simulink model "Simulation_Model_Env"  (R2024a)
settings: Solver=ode45  StartTime=0  StopTime=inf  FixedStep=0.001  MaxStep=0.1  RelTol=1e-6  AbsTol=1e-6  EnableMultiTasking=on
values from neighbouring files (symbols this model uses):
  batteryCap = 1000    [trainingData.mat]
  IrrData10pcLow = [1233 1234 1569 1570 1688 1689 4307 3623 1156 1118 1161 3247 ... (547 elements, 1x547)]    [trainingData.mat]
  pvCap = 1300    [trainingData.mat]
undefined symbols (not defined in the file or in its folder): seedDay, timeEpisode
libraries: simulink x8, rllib x1
settings Model: Creator=feliz  LastModifiedBy=bretz68
settings SolverCC: AutoScaleAbsTol=off  ZeroCrossControl=DisableAll
settings DataIOCC: LimitDataPoints=on  SaveFormat=Array
settings OptimizationCC: ExpressionDepthLimit=2147483647  LifeSpan=inf
settings DebuggingCC: UnderspecifiedInitializationDetection=Classic  MergeDetectMultiDrivingBlocksExec=none  SolverPrmCheckMsg=warning  UnconnectedInputMsg=warning  UnconnectedOutputMsg=warning  UnconnectedLineMsg=warning  AllowSymbolicDim=off  StateNameClashWarn=warning  SFUnexpectedBacktrackingDiag=warning  SFNoUnconditionalDefaultTransitionDiag=warning  SFExecutionAtInitializationDiag=none  ArithmeticOperatorsInVariantConditions=warning
settings HardwareCC: ProdBitPerPointer=32  ProdBitPerSizeT=32  ProdBitPerPtrDiffT=32  ProdLargestAtomicFloat=None  ProdIntDivRoundTo=Undefined  ProdEndianess=Unspecified  ProdWordSize=32  ProdHWDeviceType=32-bit Generic
settings ModelReferenceCC: EnableRefExpFcnMdlSchedulingChecks=on  PropagateSignalLabelsOutOfModel=off
settings SFSimCC: SimUseLocalCustomCode=off  CustomCodeUndefinedFunction=UseInterfaceOnly
settings RTWCC: RTWUseLocalCustomCode=off  GPUComputeCapability=3.5
settings CodeAppCC: StateflowObjectComments=on
settings GRTTargetCC: TargetLangStandard=C89/C90 (ANSI)
settings ConfigComp: CovMetricSettings=dw  CovSaveCumulativeToWorkspaceVar=on  CovSaveSingleToWorkspaceVar=on  CovExternalEMLEnable=off

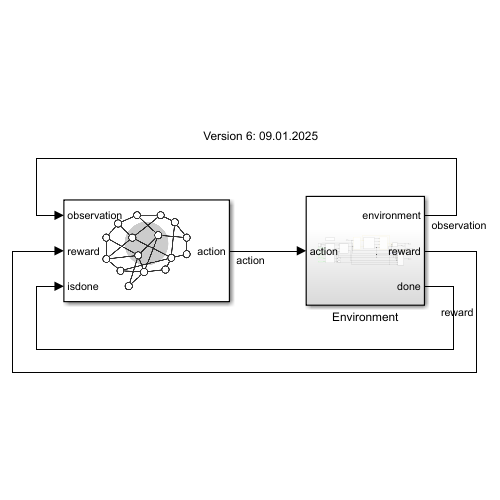
[thumbnail: Simulink's stored preview of the top-level diagram]
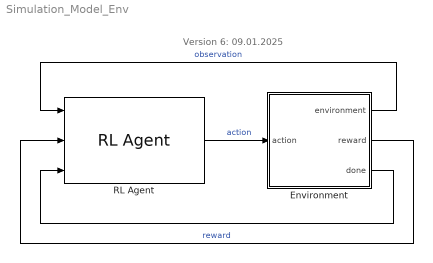
== system Simulation_Model_Env ==
  note: Version 6: 09.01.2025
  Environment : Subsystem
  RL Agent : rllib/RL Agent  Agent=ppoRealAgentv10  ExternalActionAsInput=off  ProvideLastAction=off  ProvideCumRwd=off  TreatAsDirectFeedthrough=on  UseStrictObservationDataTypes=off
  wires:
  Environment/1(environment) -> RL Agent/1  "observation"
  RL Agent/1 -> Environment/1(action)  "action"
  Environment/2(reward) -> RL Agent/2  "reward"
  Environment/3(done) -> RL Agent/3

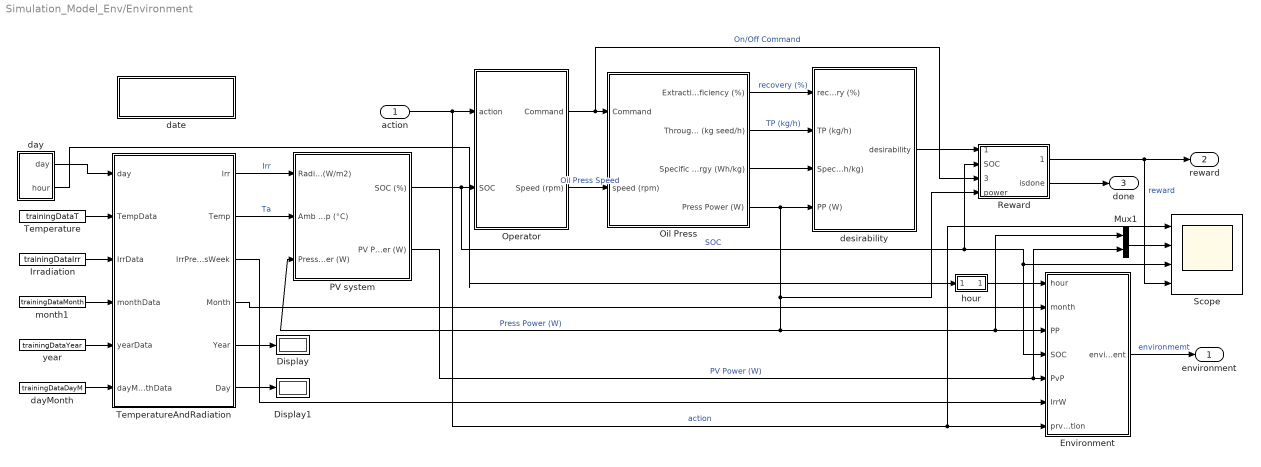
== system Simulation_Model_Env/Environment ==
  action : Inport
  Display : Display
  Display1 : Display
  Environment : Subsystem
  Irradiation : FromWorkspace  VariableName=trainingDataIrr  OutDataTypeStr=double  SampleTime=timeEpisode+1
  Mux1 : Mux  Inputs=2
  Oil Press : Subsystem
  Operator : Subsystem
  PV system : Subsystem
  Reward : Subsystem
  Scope : Scope  NumInputPorts=4
  Temperature : FromWorkspace  VariableName=trainingDataT  OutDataTypeStr=double  SampleTime=timeEpisode+1
  TemperatureAndRadiation : MATLAB Function  TreatAsAtomicUnit=on
  date : Subsystem
  day : Subsystem
  dayMonth : FromWorkspace  VariableName=trainingDataDayM  OutDataTypeStr=double  SampleTime=timeEpisode+1
  desirability : Subsystem
  hour : Subsystem
  month1 : FromWorkspace  VariableName=trainingDataMonth  OutDataTypeStr=double  SampleTime=timeEpisode+1
  year : FromWorkspace  VariableName=trainingDataYear  OutDataTypeStr=double  SampleTime=timeEpisode+1
  environment : Outport
  reward : Outport  Port=2
  done : Outport  Port=3
  wires:
  TemperatureAndRadiation/2(Temp) -> PV system/2(Amb Temp (°C))  "Ta"
  Operator/1("Command ") -> Reward/3(command), Oil Press/1(Command)  "On/Off Command"
  Irradiation/1 -> TemperatureAndRadiation/3(IrrData)
  TemperatureAndRadiation/1(Irr) -> PV system/1(Radiation on Surf (W/m2))  "Irr"
  Temperature/1 -> TemperatureAndRadiation/2(TempData)
  Oil Press/2(Throughput (kg seed/h)) -> desirability/2(TP (kg/h))  "TP (kg/h)"
  Operator/2(Speed (rpm)) -> Oil Press/2(speed (rpm))  "Oil Press Speed"
  Oil Press/1(Extraction Efficiency (%)) -> desirability/1(recovery (%))  "recovery (%)"
  desirability/1(desirability) -> Reward/1(desirability)
  Oil Press/3(Specific energy (Wh/kg)) -> desirability/3(Spec Enr (Wh/kg))
  TemperatureAndRadiation/3(IrrPreviousWeek) -> Environment/6(IrrW)
  hour/1(hour) -> Environment/1(hour)
  day/1(day) -> TemperatureAndRadiation/1(day)
  Reward/2(isdone) -> done/1
  Environment/1(environment) -> environment/1  "environmemt"
  month1/1 -> TemperatureAndRadiation/4(monthData)
  TemperatureAndRadiation/4(Month) -> Environment/2(month)
  PV system/1(SOC (%)) -> Environment/4(SOC), Scope/3, Reward/2(SOC), Operator/2(SOC)  "SOC"
  Mux1/1 -> Scope/2
  action/1 -> Operator/1(action), Environment/7(prvAction), Scope/1  "action"
  Reward/1(reward) -> Scope/4, reward/1  "reward"
  Oil Press/4("Press Power (W) ") -> desirability/4(PP (W)), Reward/4(power), Environment/3(PP), Mux1/1, PV system/3(Press Power (W))  "Press Power (W)"
  PV system/2(PV Power (W)) -> Mux1/2, Environment/5(PvP)  "PV Power (W)"
  year/1 -> TemperatureAndRadiation/5(yearData)
  TemperatureAndRadiation/5(Year) -> Display/1
  TemperatureAndRadiation/6(Day) -> Display1/1
  dayMonth/1 -> TemperatureAndRadiation/6(dayMonthData)
  day/2(hour) -> hour/1(simhour)

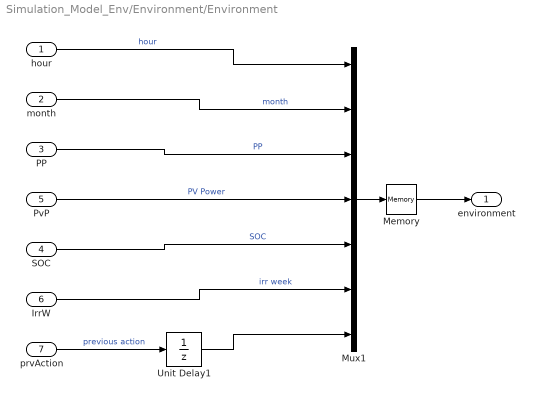
== system Simulation_Model_Env/Environment/Environment ==
  hour : Inport
  month : Inport  Port=2
  PP : Inport  Port=3
  SOC : Inport  Port=4
  PvP : Inport  Port=5
  IrrW : Inport  Port=6
  prvAction : Inport  Port=7
  Memory : Memory
  Mux1 : Mux  Inputs=7
  Unit Delay1 : UnitDelay  SampleTime=-1  HasFrameUpgradeWarning=on
  environment : Outport
  wires:
  SOC/1 -> Mux1/5  "SOC"
  PvP/1 -> Mux1/4  "PV Power"
  IrrW/1 -> Mux1/6  "irr week"
  hour/1 -> Mux1/1  "hour"
  PP/1 -> Mux1/3  "PP"
  month/1 -> Mux1/2  "month"
  Mux1/1 -> Memory/1
  prvAction/1 -> Unit Delay1/1  "previous action"
  Unit Delay1/1 -> Mux1/7
  Memory/1 -> environment/1

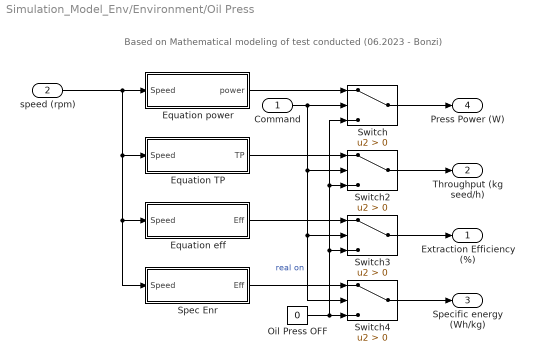
== system Simulation_Model_Env/Environment/Oil Press ==
  note: Based on Mathematical modeling of test conducted (06.2023 - Bonzi)
  Command : Inport
  speed (rpm) : Inport  Port=2
  Equation TP : Subsystem
  Equation eff : Subsystem
  Equation power : Subsystem
  Oil Press OFF : Constant  Value=0
  Spec Enr : Subsystem
  Switch{,2..4} (4 alike) : Switch  Criteria=u2 > Threshold  SaturateOnIntegerOverflow=off  InputSameDT=off
  Extraction Efficiency (%) : Outport
  Throughput (kg seed/h) : Outport  Port=2
  Specific energy (Wh/kg) : Outport  Port=3
  "Press Power (W) " : Outport  Port=4
  wires:
  Switch3/1 -> Extraction Efficiency (%)/1
  Switch/1 -> "Press Power (W) "/1
  Equation power/1(power) -> Switch/1
  Equation TP/1(TP) -> Switch2/1
  Switch2/1 -> Throughput (kg seed/h)/1
  Equation eff/1(Eff) -> Switch3/1
  Oil Press OFF/1 -> Switch3/3, Switch2/3, Switch/3, Switch4/3
  speed (rpm)/1 -> Spec Enr/1(Speed), Equation eff/1(Speed), Equation TP/1(Speed), Equation power/1(Speed)
  Command/1 -> Switch4/2, Switch3/2, Switch2/2, Switch/2  "real on"
  Switch4/1 -> Specific energy (Wh/kg)/1
  Spec Enr/1(Eff) -> Switch4/1

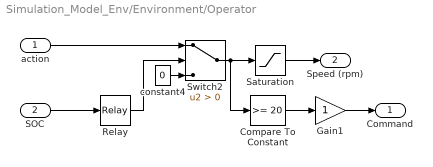
== system Simulation_Model_Env/Environment/Operator ==
  action : Inport
  SOC : Inport  Port=2
  Compare To Constant : simulink/Logic and Bit Operations/Compare To Constant  relop=>=  const=20  OutDataTypeStr=boolean
  Gain1 : Gain  OutDataTypeStr=double
  Relay : Relay  OnSwitchValue=25  OffSwitchValue=20
  Saturation : Saturate  UpperLimit=70  LowerLimit=0
  Switch2 : Switch  Criteria=u2 > Threshold  SaturateOnIntegerOverflow=off  InputSameDT=off
  constant4 : Constant  Value=0
  "Command " : Outport
  Speed (rpm) : Outport  Port=2
  wires:
  SOC/1 -> Relay/1
  Switch2/1 -> Compare To Constant/1, Saturation/1
  Relay/1 -> Switch2/2
  action/1 -> Switch2/1
  constant4/1 -> Switch2/3
  Compare To Constant/1 -> Gain1/1
  Saturation/1 -> Speed (rpm)/1
  Gain1/1 -> "Command "/1

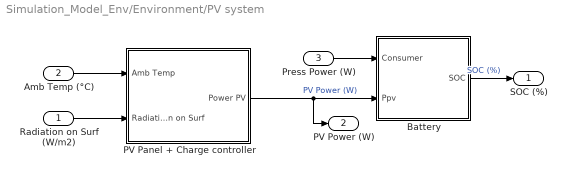
== system Simulation_Model_Env/Environment/PV system ==
  Radiation on Surf (W/m2) : Inport
  Amb Temp (°C) : Inport  Port=2
  Press Power (W) : Inport  Port=3
  Battery : Subsystem
      mask Display: image('bat.PNG'); % Use "Edit Image" on toolstrip to change.
  PV Panel + Charge controller : Subsystem
      mask Display: image('pvmppt.PNG'); % Use "Edit Image" on toolstrip to change.
  SOC (%) : Outport
  PV Power (W) : Outport  Port=2
  wires:
  Amb Temp (°C)/1 -> PV Panel + Charge controller/1(Amb Temp)
  PV Panel + Charge controller/1(Power PV) -> PV Power (W)/1, Battery/2(Ppv)  "PV Power (W)"
  Press Power (W)/1 -> Battery/1(Consumer)
  Battery/1(SOC) -> SOC (%)/1  "SOC (%)"
  Radiation on Surf (W/m2)/1 -> PV Panel + Charge controller/2(Radiation on Surf)

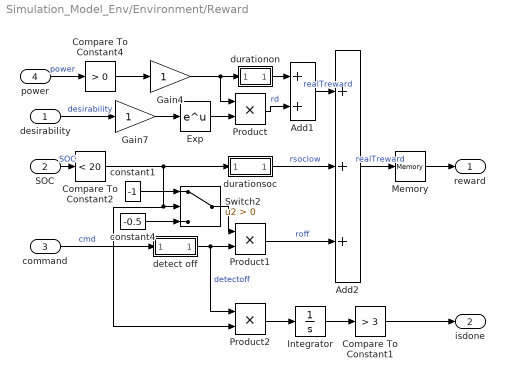
== system Simulation_Model_Env/Environment/Reward ==
  desirability : Inport
  SOC : Inport  Port=2
  command : Inport  Port=3
  power : Inport  Port=4
  Add1 : Sum
  Add2 : Sum  Inputs=+++
  Compare To Constant1 : simulink/Logic and Bit Operations/Compare To Constant  relop=>  const=3  OutDataTypeStr=boolean
  Compare To Constant2 : simulink/Logic and Bit Operations/Compare To Constant  relop=<  const=20  OutDataTypeStr=boolean
  Compare To Constant4 : simulink/Logic and Bit Operations/Compare To Constant  relop=>  const=0  OutDataTypeStr=boolean
  Exp : Math
  Gain4 : Gain  OutDataTypeStr=double
  Gain7 : Gain  OutDataTypeStr=double
  Integrator : Integrator
  Memory : Memory
  Product : Product
  Product1 : Product
  Product2 : Product  OutDataTypeStr=double
  Switch2 : Switch  Criteria=u2 > Threshold  SaturateOnIntegerOverflow=off  InputSameDT=off
  constant1 : Constant  Value=-1
  constant4 : Constant  Value=-0.5
  detect off : Subsystem
  durationon : Subsystem
  durationsoc : Subsystem
  reward : Outport
  isdone : Outport  Port=2
  wires:
  desirability/1 -> Gain7/1  "desirability"
  Gain7/1 -> Exp/1
  durationsoc/1(Out1) -> Add2/2  "rsoclow"
  Add2/1 -> Memory/1  "realTreward"
  Exp/1 -> Product/2
  Memory/1 -> reward/1
  detect off/1(Out1) -> Product2/1, Product1/2  "detectoff"
  command/1 -> detect off/1(cmd)  "cmd"
  Product1/1 -> Add2/3  "roff"
  SOC/1 -> Compare To Constant2/1  "SOC"
  Compare To Constant4/1 -> Gain4/1
  Gain4/1 -> durationon/1(on), Product/1
  Product/1 -> Add1/2  "rd"
  constant4/1 -> Switch2/3
  constant1/1 -> Switch2/1
  Switch2/1 -> Product1/1
  power/1 -> Compare To Constant4/1  "power"
  Compare To Constant2/1 -> durationsoc/1(isco), Product2/2, Switch2/2
  Add1/1 -> Add2/1  "realTreward"
  durationon/1(Out1) -> Add1/1
  Integrator/1 -> Compare To Constant1/1
  Compare To Constant1/1 -> isdone/1
  Product2/1 -> Integrator/1

== system Simulation_Model_Env/Environment/date ==
  note: /
  note: Date
  note: /
  Display1 : DisplayBlock  LabelPosition=Hide  Transparency=1
  Display2 : DisplayBlock  LabelPosition=Hide  Transparency=1  ShowGrid=off
  Display3 : DisplayBlock  LabelPosition=Hide  Transparency=1  ShowGrid=off

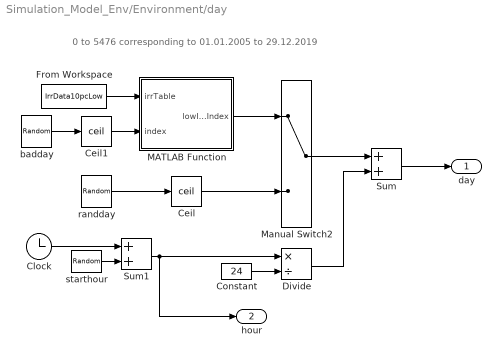
== system Simulation_Model_Env/Environment/day ==
  note: 0 to 5476 corresponding to 01.01.2005 to 29.12.2019
  Ceil : Rounding  Operator=ceil
  Ceil1 : Rounding  Operator=ceil
  Clock : Clock
  Constant : Constant  Value=24
  Divide : Product  Inputs=*/
  From Workspace : FromWorkspace  VariableName=IrrData10pcLow  SampleTime=timeEpisode+1
  MATLAB Function : MATLAB Function  TreatAsAtomicUnit=on
  Manual Switch2 : ManualSwitch
  Sum : Sum
  Sum1 : Sum
  badday : UniformRandomNumber  Minimum=0  Maximum=length(IrrData10pcLow)-1  Seed=seedDay  SampleTime=timeEpisode+1
  randday : UniformRandomNumber  Minimum=0  Maximum=5476  Seed=seedDay  SampleTime=timeEpisode+1
  starthour : UniformRandomNumber  Minimum=0  Maximum=23  Seed=seedDay  SampleTime=timeEpisode+1
  day : Outport
  hour : Outport  Port=2
  wires:
  randday/1 -> Ceil/1
  Ceil/1 -> Manual Switch2/2
  Constant/1 -> Divide/2
  Clock/1 -> Sum1/1
  Divide/1 -> Sum/2
  Sum/1 -> day/1
  From Workspace/1 -> MATLAB Function/1(irrTable)
  MATLAB Function/1(lowIrrDayIndex) -> Manual Switch2/1
  Manual Switch2/1 -> Sum/1
  starthour/1 -> Sum1/2
  Sum1/1 -> hour/1, Divide/1
  badday/1 -> Ceil1/1
  Ceil1/1 -> MATLAB Function/2(index)

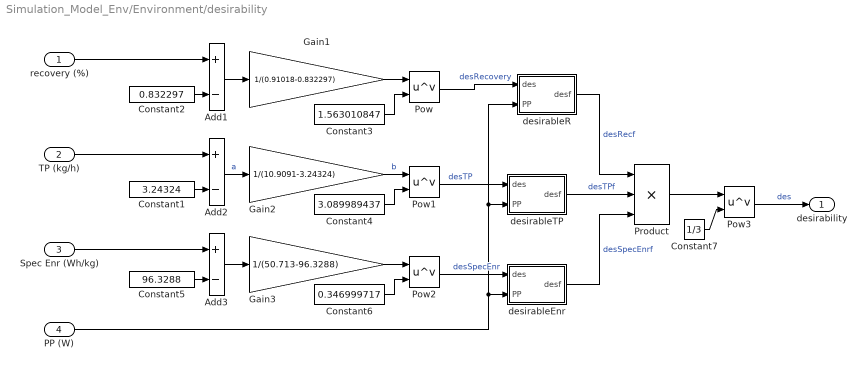
== system Simulation_Model_Env/Environment/desirability ==
  recovery (%) : Inport
  TP (kg/h) : Inport  Port=2
  Spec Enr (Wh/kg) : Inport  Port=3
  PP (W) : Inport  Port=4
  Add1 : Sum  Inputs=+-
  Add2 : Sum  Inputs=+-
  Add3 : Sum  Inputs=+-
  Constant1 : Constant  Value=3.24324
  Constant2 : Constant  Value=0.832297
  Constant3 : Constant  Value=1.563010847
  Constant4 : Constant  Value=3.089989437
  Constant5 : Constant  Value=96.3288
  Constant6 : Constant  Value=0.346999717
  Constant7 : Constant  Value=1/3
  Gain1 : Gain  Gain=1/(0.91018-0.832297)
  Gain2 : Gain  Gain=1/(10.9091-3.24324)
  Gain3 : Gain  Gain=1/(50.713-96.3288)
  Pow{,1..3} (4 alike) : Math  Operator=pow  SignedPower=on  RndMeth=Zero
  Product : Product  Inputs=3
  desirableEnr : Subsystem
  desirableR : Subsystem
  desirableTP : Subsystem
  desirability : Outport
  wires:
  Add1/1 -> Gain1/1
  recovery (%)/1 -> Add1/1
  Constant2/1 -> Add1/2
  Gain1/1 -> Pow/1
  Constant3/1 -> Pow/2
  Constant1/1 -> Add2/2
  Gain2/1 -> Pow1/1  "b"
  Constant4/1 -> Pow1/2
  Add2/1 -> Gain2/1  "a"
  TP (kg/h)/1 -> Add2/1
  Add3/1 -> Gain3/1
  Gain3/1 -> Pow2/1
  Constant5/1 -> Add3/2
  Constant6/1 -> Pow2/2
  Spec Enr (Wh/kg)/1 -> Add3/1
  Product/1 -> Pow3/1
  desirableTP/1(desf) -> Product/2  "desTPf"
  desirableEnr/1(desf) -> Product/3  "desSpecEnrf"
  Pow/1 -> desirableR/1(des)  "desRecovery"
  desirableR/1(desf) -> Product/1  "desRecf"
  Pow1/1 -> desirableTP/1(des)  "desTP"
  Pow2/1 -> desirableEnr/1(des)  "desSpecEnr"
  PP (W)/1 -> desirableR/2(PP), desirableTP/2(PP), desirableEnr/2(PP)
  Constant7/1 -> Pow3/2
  Pow3/1 -> desirability/1  "des"

== system Simulation_Model_Env/Environment/hour ==
  simhour : Inport
  Constant : Constant  Value=24
  Mod : Math  Operator=mod
  hour : Outport
  wires:
  simhour/1 -> Mod/1
  Mod/1 -> hour/1
  Constant/1 -> Mod/2

== system Simulation_Model_Env/Environment/Oil Press/Equation TP ==
  Speed : Inport
  Add : Sum  Inputs=+++
  Gain1 : Gain  Gain=0.217737397
  Product : Product  Inputs=3
  constant : Constant  Value=-0.000675351
  constant4 : Constant  Value=-0.998344774
  TP : Outport
  wires:
  Gain1/1 -> Add/2
  Product/1 -> Add/3
  constant/1 -> Product/3
  constant4/1 -> Add/1
  Speed/1 -> Gain1/1, Product/2, Product/1
  Add/1 -> TP/1

== system Simulation_Model_Env/Environment/Oil Press/Equation eff ==
  Speed : Inport
  Add : Sum  Inputs=+++
  Gain1 : Gain  Gain=-0.003110656
  Product : Product  Inputs=3
  constant : Constant  Value=2.56866E-05
  constant4 : Constant  Value=0.95370599
  Eff : Outport
  wires:
  Gain1/1 -> Add/2
  Product/1 -> Add/3
  constant/1 -> Product/3
  constant4/1 -> Add/1
  Speed/1 -> Product/2, Product/1, Gain1/1
  Add/1 -> Eff/1

== system Simulation_Model_Env/Environment/Oil Press/Equation power ==
  Speed : Inport
  Add : Sum  Inputs=+++
  Gain1 : Gain  Gain=8.7
  Product : Product  Inputs=3
  constant : Constant  Value=-0.05
  constant4 : Constant  Value=57.3
  power : Outport
  wires:
  Gain1/1 -> Add/2
  Product/1 -> Add/3
  constant/1 -> Product/3
  constant4/1 -> Add/1
  Speed/1 -> Gain1/1, Product/2, Product/1
  Add/1 -> power/1

== system Simulation_Model_Env/Environment/Oil Press/Spec Enr ==
  Speed : Inport
  Add : Sum  Inputs=+++
  Gain1 : Gain  Gain=-0.977028804
  Product : Product  Inputs=3
  constant : Constant  Value=0.004169482
  constant4 : Constant  Value=97.14879537
  Eff : Outport
  wires:
  Gain1/1 -> Add/2
  Product/1 -> Add/3
  constant/1 -> Product/3
  constant4/1 -> Add/1
  Speed/1 -> Product/2, Product/1, Gain1/1
  Add/1 -> Eff/1

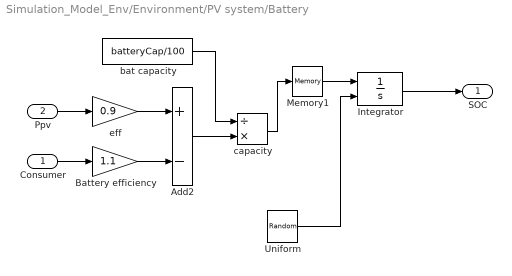
== system Simulation_Model_Env/Environment/PV system/Battery ==
  Consumer : Inport
  Ppv : Inport  Port=2
  Add2 : Sum  Inputs=+-
  Battery efficiency : Gain  Gain=1.1
  Integrator : Integrator  InitialConditionSource=external  InitialCondition=20  LimitOutput=on  UpperSaturationLimit=100  LowerSaturationLimit=0
  Memory1 : Memory
  Uniform : UniformRandomNumber  Minimum=20  Maximum=100  Seed=seedDay  SampleTime=timeEpisode+1
  bat capacity : Constant  Value=batteryCap/100
  capacity : Product  Inputs=/*
  eff : Gain  Gain=0.9
  SOC : Outport
  wires:
  Ppv/1 -> eff/1
  Consumer/1 -> Battery efficiency/1
  capacity/1 -> Memory1/1
  Add2/1 -> capacity/2
  bat capacity/1 -> capacity/1
  eff/1 -> Add2/1
  Battery efficiency/1 -> Add2/2
  Integrator/1 -> SOC/1
  Uniform/1 -> Integrator/2
  Memory1/1 -> Integrator/1

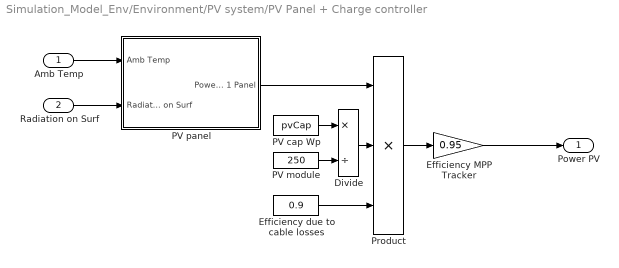
== system Simulation_Model_Env/Environment/PV system/PV Panel + Charge controller ==
  Amb Temp : Inport
  Radiation on Surf : Inport  Port=2
  Divide : Product  Inputs=*/
  Efficiency MPP Tracker : Gain  Gain=0.95
  Efficiency due to cable losses : Constant  Value=0.9
  PV cap Wp : Constant  Value=pvCap
  PV module : Constant  Value=250
  PV panel : Subsystem
  Product : Product  Inputs=3  RndMeth=Zero
  Power PV : Outport
  wires:
  Product/1 -> Efficiency MPP Tracker/1
  Efficiency MPP Tracker/1 -> Power PV/1
  PV panel/1(Power PV 1 Panel) -> Product/1
  PV cap Wp/1 -> Divide/1
  Efficiency due to cable losses/1 -> Product/3
  Amb Temp/1 -> PV panel/1(Amb Temp)
  Radiation on Surf/1 -> PV panel/2(Radiation on Surf)
  Divide/1 -> Product/2
  PV module/1 -> Divide/2

== system Simulation_Model_Env/Environment/Reward/detect off ==
  cmd : Inport
  Add : Sum  Inputs=+-
  Compare To Constant : simulink/Logic and Bit Operations/Compare To Constant  relop=<  const=0  OutDataTypeStr=boolean
  Unit Delay : UnitDelay  SampleTime=-1  HasFrameUpgradeWarning=on
  Out1 : Outport
  wires:
  Add/1 -> Compare To Constant/1
  Unit Delay/1 -> Add/2  "cmdDel"
  cmd/1 -> Unit Delay/1, Add/1  "cmd"
  Compare To Constant/1 -> Out1/1  "intdiff"

== system Simulation_Model_Env/Environment/Reward/durationon ==
  on : Inport
  Add : Sum
  Gain3 : Gain  Gain=0.01  OutDataTypeStr=double
  Memory : Memory
  Product : Product
  Out1 : Outport
  wires:
  Add/1 -> Product/2
  Memory/1 -> Add/2
  Gain3/1 -> Add/1
  on/1 -> Product/1, Gain3/1
  Product/1 -> Memory/1, Out1/1

== system Simulation_Model_Env/Environment/Reward/durationsoc ==
  isco : Inport
  Add : Sum
  Gain1 : Gain  Gain=-1  OutDataTypeStr=double
  Gain3 : Gain  Gain=0.02  OutDataTypeStr=double
  Memory : Memory
  Product : Product
  Out1 : Outport
  wires:
  Add/1 -> Product/2
  Memory/1 -> Add/2
  Gain3/1 -> Add/1
  Product/1 -> Memory/1, Gain1/1
  isco/1 -> Product/1, Gain3/1
  Gain1/1 -> Out1/1  "rsoclow"

== system Simulation_Model_Env/Environment/desirability/desirableEnr ==
  des : Inport
  PP : Inport  Port=2
  Compare To Constant : simulink/Logic and Bit Operations/Compare To Constant  relop=>  const=0  OutDataTypeStr=boolean
  Product : Product
  Saturation : Saturate  UpperLimit=1  LowerLimit=0
  desf : Outport
  wires:
  des/1 -> Saturation/1
  Product/1 -> desf/1
  Saturation/1 -> Product/1
  PP/1 -> Compare To Constant/1
  Compare To Constant/1 -> Product/2

== system Simulation_Model_Env/Environment/desirability/desirableR ==
  des : Inport
  PP : Inport  Port=2
  Compare To Constant : simulink/Logic and Bit Operations/Compare To Constant  relop=>  const=0  OutDataTypeStr=boolean
  Product : Product
  Saturation : Saturate  UpperLimit=1  LowerLimit=0
  desf : Outport
  wires:
  des/1 -> Saturation/1
  Saturation/1 -> Product/1
  PP/1 -> Compare To Constant/1
  Product/1 -> desf/1
  Compare To Constant/1 -> Product/2

== system Simulation_Model_Env/Environment/desirability/desirableTP ==
  des : Inport
  PP : Inport  Port=2
  Compare To Constant : simulink/Logic and Bit Operations/Compare To Constant  relop=>  const=0  OutDataTypeStr=boolean
  Product : Product
  Saturation : Saturate  UpperLimit=1  LowerLimit=0
  desf : Outport
  wires:
  des/1 -> Saturation/1
  Product/1 -> desf/1
  Saturation/1 -> Product/1
  PP/1 -> Compare To Constant/1
  Compare To Constant/1 -> Product/2  "a"

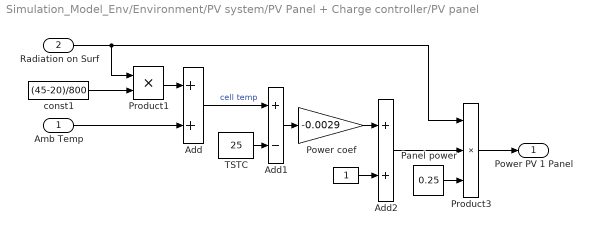
== system Simulation_Model_Env/Environment/PV system/PV Panel + Charge controller/PV panel ==
  Amb Temp : Inport
  Radiation on Surf : Inport  Port=2
  " " : Constant
  Add : Sum
  Add1 : Sum  Inputs=+-
  Add2 : Sum
  Panel power : Constant  Value=0.25
  Power coef : Gain  Gain=-0.0029
  Product1 : Product  RndMeth=Zero
  Product3 : Product  Inputs=3  RndMeth=Zero
  TSTC : Constant  Value=25
  const1 : Constant  Value=(45-20)/800
  Power PV 1 Panel : Outport
  wires:
  Amb Temp/1 -> Add/2
  Radiation on Surf/1 -> Product3/1, Product1/1
  Add/1 -> Add1/1  "cell temp"
  Product1/1 -> Add/1
  const1/1 -> Product1/2
  Product3/1 -> Power PV 1 Panel/1
  TSTC/1 -> Add1/2
  Add1/1 -> Power coef/1
  " "/1 -> Add2/2
  Power coef/1 -> Add2/1
  Add2/1 -> Product3/2
  Panel power/1 -> Product3/3

== matlab function Simulation_Model_Env/Environment/TemperatureAndRadiation ==
  data: day input; TempData input; IrrData input; Irr output; Temp output; IrrPreviousWeek output; monthData input; Month output; yearData input; Year output; dayMonthData input; Day output
function [Irr, Temp, IrrPreviousWeek, Month, Year, Day] = fcn(day, TempData,IrrData, monthData, yearData, dayMonthData)
index=1+(day-1)*24;

Irr = interp1(IrrData,index);
Temp = interp1(TempData,index);
Month = interp1(monthData,index);
Year = interp1(yearData,index);
Day = round(interp1(dayMonthData,index));

iniPreviousWeek=max(1+(ceil(day)-8)*24,1);
finiPreviousWeek=min((ceil(day)-1)*24+23,(5479)*24);

IrrPreviousWeek=mean(IrrData(iniPreviousWeek:finiPreviousWeek));
end

== matlab function Simulation_Model_Env/Environment/day/MATLAB Function ==
  data: irrTable input; lowIrrDayIndex output; index input
function lowIrrDayIndex = fcn(irrTable, index)

    % Get the value from the table using the random index
    lowIrrDayIndex = irrTable(index);

end
